simulink model "MyTwoTankSystem"  (R2021b)
settings: Solver=ode4  StartTime=0.0  StopTime=SIM_TIME  FixedStep=STEP_SIZE  RelTol=1e-3  EnableMultiTasking=on
undefined symbols (not defined in the file): At, C0, Dv, ka, kh, kt, u10, u20, v10, v20, v30, x0
settings Model: Creator=tanzc  LastModifiedBy=tanzc
settings DataIOCC: InitialState=x0  LimitDataPoints=on  SaveFinalState=on  SaveFormat=Array  ReturnWorkspaceOutputs=off

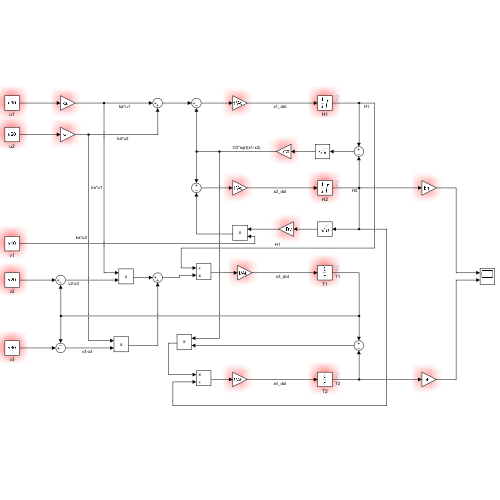
[thumbnail: Simulink's stored preview of the top-level diagram]
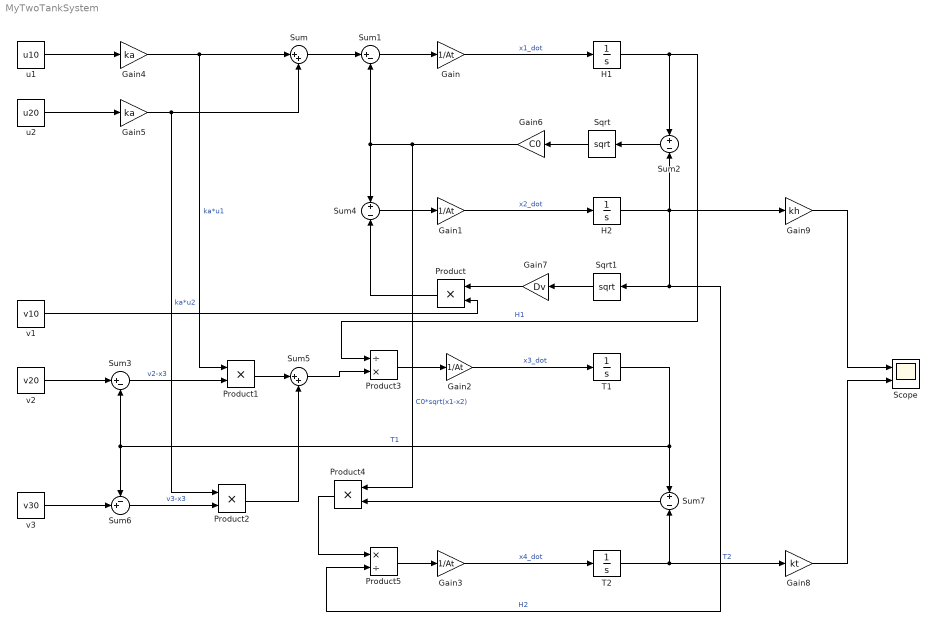
== system MyTwoTankSystem ==
  Gain{,1..3} (4 alike) : Gain  Gain=1/At
  Gain4 : Gain  Gain=ka
  Gain5 : Gain  Gain=ka
  Gain6 : Gain  Gain=C0
  Gain7 : Gain  Gain=Dv
  Gain8 : Gain  Gain=kt
  Gain9 : Gain  Gain=kh
  H1 : Integrator  Priority=1  InitialCondition=x0(1)  LimitOutput=on  LowerSaturationLimit=0
  H2 : Integrator  Priority=2  InitialCondition=x0(2)  LimitOutput=on  LowerSaturationLimit=0
  Product{,1..2,4} (4 alike) : Product
  Product3 : Product  Inputs=/*
  Product5 : Product  Inputs=*/
  Scope : Scope  NumInputPorts=2
  Sqrt : Sqrt  SaturateOnIntegerOverflow=on
  Sqrt1 : Sqrt  SaturateOnIntegerOverflow=on
  Sum : Sum  Inputs=|++
  Sum1 : Sum  Inputs=|+-
  Sum2 : Sum  Inputs=+-
  Sum3 : Sum  Inputs=|+-
  Sum4 : Sum  Inputs=+-
  Sum5 : Sum  Inputs=|++
  Sum6 : Sum  Inputs=-+|
  Sum7 : Sum  Inputs=+-
  T1 : Integrator  Priority=3  InitialCondition=x0(3)
  T2 : Integrator  Priority=4  InitialCondition=x0(4)
  u1 : Constant  Value=u10
  u2 : Constant  Value=u20
  v1 : Constant  Value=v10
  v2 : Constant  Value=v20
  v3 : Constant  Value=v30
  wires:
  H1/1 -> Sum2/1, Product3/1  "H1"
  Gain/1 -> H1/1  "x1_dot"
  H2/1 -> Gain9/1, Product5/2, Sqrt1/1, Sum2/2  "H2"
  Gain1/1 -> H2/1  "x2_dot"
  T1/1 -> Sum3/2, Sum6/1, Sum7/1  "T1"
  Gain2/1 -> T1/1  "x3_dot"
  T2/1 -> Gain8/1, Sum7/2  "T2"
  Gain3/1 -> T2/1  "x4_dot"
  u1/1 -> Gain4/1
  u2/1 -> Gain5/1
  Gain4/1 -> Product1/1, Sum/1  "ka*u1"
  Gain5/1 -> Product2/1, Sum/2  "ka*u2"
  Sum/1 -> Sum1/1
  Sum1/1 -> Gain/1
  Sum2/1 -> Sqrt/1
  Sqrt/1 -> Gain6/1
  Gain6/1 -> Sum4/1, Sum1/2, Product4/1  "C0*sqrt(x1-x2)"
  Sqrt1/1 -> Gain7/1
  v1/1 -> Product/2
  Gain7/1 -> Product/1
  Product/1 -> Sum4/2
  Sum4/1 -> Gain1/1
  v2/1 -> Sum3/1
  Sum3/1 -> Product1/2  "v2-x3"
  v3/1 -> Sum6/2
  Sum6/1 -> Product2/2  "v3-x3"
  Product2/1 -> Sum5/2
  Product1/1 -> Sum5/1
  Sum5/1 -> Product3/2
  Product3/1 -> Gain2/1
  Sum7/1 -> Product4/2
  Product5/1 -> Gain3/1
  Product4/1 -> Product5/1
  Gain9/1 -> Scope/1
  Gain8/1 -> Scope/2
